simulink model "exact_lin_control"  (R2017a)
settings: Solver=VariableStepAuto  StartTime=0.0  StopTime=10  RelTol=1e-3
undefined symbols (not defined in the file or in its folder): controlfun, K, plantfun, transfsfun, x0
settings Model: Creator=bruno  LastModifiedBy=bruno

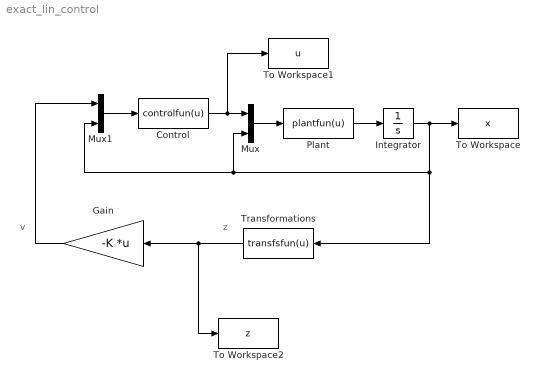
== system exact_lin_control ==
  note: z
  note: v
  "Control " : MATLABFcn  MATLABFcn=controlfun(u)  OutputSignalType=real
  Gain : Gain  Gain=-K  Multiplication=Matrix(K*u) (u vector)
  Integrator : Integrator  InitialCondition=x0
  Mux : Mux  Inputs=2
  Mux1 : Mux  Inputs=2
  Plant : MATLABFcn  MATLABFcn=plantfun(u)  OutputSignalType=real
  To Workspace : ToWorkspace  VariableName=x  SaveFormat=Timeseries  SampleTime=-1
  To Workspace1 : ToWorkspace  VariableName=u  SaveFormat=Timeseries  SampleTime=-1
  To Workspace2 : ToWorkspace  VariableName=z  SaveFormat=Timeseries  SampleTime=-1
  Transformations : MATLABFcn  MATLABFcn=transfsfun(u)  OutputSignalType=real
  wires:
  Plant/1 -> Integrator/1
  Integrator/1 -> Mux/2, Mux1/2, Transformations/1, To Workspace/1
  Mux/1 -> Plant/1
  "Control "/1 -> To Workspace1/1, Mux/1
  Transformations/1 -> To Workspace2/1, Gain/1
  Mux1/1 -> "Control "/1
  Gain/1 -> Mux1/1
